simulink model "Bai22"  (R2015a)
settings: Solver=ode45  StartTime=0.0  StopTime=10.0  RelTol=1e-3
libraries: commchan3 x1, simulink x1
settings Model: Creator=Win 10  LastModifiedBy=Win 10

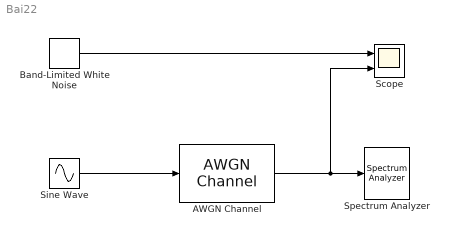
== system Bai22 ==
  AWGN Channel : commchan3/AWGN Channel  InputProcessing=Columns as channels (frame based)  seed=67  noiseMode=Variance from mask  EbNodB=10  EsNodB=10  SNRdB=10  bitsPerSym=1  Ps=1  Tsym=1  variance=0.5
  Band-Limited White Noise : simulink/Sources/Band-Limited White Noise  Cov=[1e-8]  Ts=1/1000  seed=[23341]  VectorParams1D=off
  Scope : Scope  NumInputPorts=2
      settings: YMin=-5~-5  YMax=5~5
  Sine Wave : Sin  Frequency=10000000  SampleTime=1/1000
  Spectrum Analyzer : SpectrumAnalyzer
  wires:
  Band-Limited White Noise/1 -> Scope/1
  AWGN Channel/1 -> Scope/2, Spectrum Analyzer/1
  Sine Wave/1 -> AWGN Channel/1
